simulink model "IC_HW4_Q4"  (R2022b)
settings: Solver=FixedStepAuto  StartTime=0.0  StopTime=SimTime  FixedStep=Delta_t  RelTol=1e-6
values from neighbouring files (symbols this model uses):
  g = 9.81    [aero_guid_dat.m]
  Iyy = 182.5/(Kg2slug*m2ft^2)    (= 247.436636441)    [aero_guid_dat.m]
  L = 0.0065    [aero_guid_dat.m]
undefined symbols (not defined in the file or in its folder): AF, c, Delta_t, Dis, IC, Ixx, Izz, lambda, m, magnitude, N_n, Out_sampleTime, Unc
settings Model: PacingRate=1.400000  Creator=Mahdi  LastModifiedBy=Mahdi
settings OptimizationCC: UseDivisionForNetSlopeComputation=on  GainParamInheritBuiltInType=on  UseFloatMulNetSlope=on  EnhancedBackFolding=on  PassReuseOutputArgsThreshold=0  MaxStackSize=64  OptimizeBlockOrder=speed  DifferentSizesBufferReuse=on
settings DebuggingCC: MultiTaskRateTransMsg=warning  ParameterTunabilityLossMsg=error  UnconnectedInputMsg=warning  UnconnectedOutputMsg=warning  UnconnectedLineMsg=warning
settings ModelReferenceCC: EnableRefExpFcnMdlSchedulingChecks=on
settings SFSimCC: MATLABDynamicMemAlloc=off
settings RTWCC: GenerateReport=on  BuildConfiguration=Faster Runs  LaunchReport=on  DLArmComputeVersion=19.05
settings CodeAppCC: ForceParamTrailComments=on  OperatorAnnotations=on  StateflowObjectComments=on
settings GRTTargetCC: TargetLangStandard=C89/C90 (ANSI)

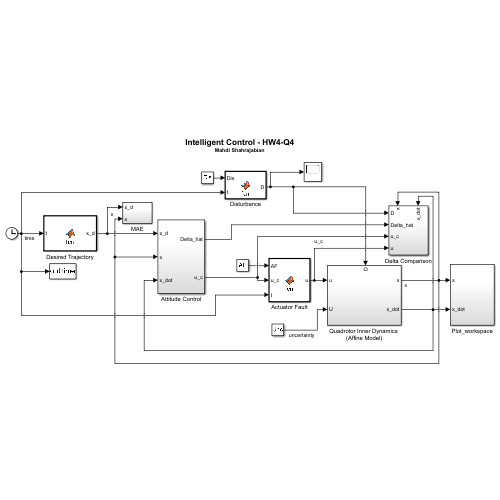
[thumbnail: Simulink's stored preview of the top-level diagram]
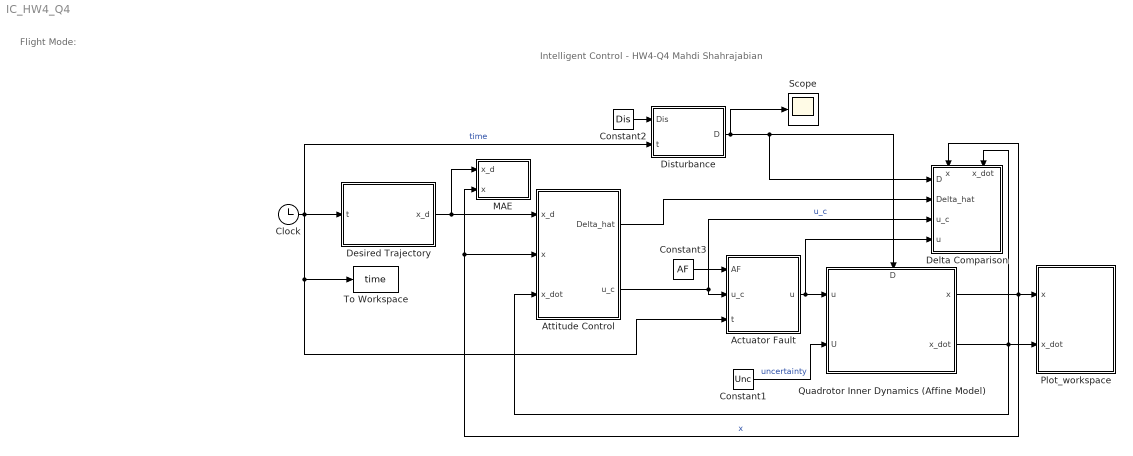
== system IC_HW4_Q4 ==
  note: Flight Mode:
  note: Intelligent Control - HW4-Q4
      | Mahdi Shahrajabian
  Actuator Fault : MATLAB Function  TreatAsAtomicUnit=on
  Attitude Control : Subsystem
  Clock : Clock
  Constant1 : Constant  Value=Unc
  Constant2 : Constant  Value=Dis
  Constant3 : Constant  Value=AF
  Delta Comparison : Subsystem
      settings: PortSchema="{\"entries\":[{\"content\":{\"sides\":[{\"content\":{\"connectorIds\":[\"In1\",\"In2\",\"In3\",\"In4\"]},\"type\":\"ConnectorPlacement.EquallySpacedRectSide\",\"uuid\":\"cdb532f7-5b91-47b5-acb3-9a86cd5c6b77\"},{\"content\":{\"connectorIds\":[],\"side\":\"RIGHT\"},\"type\":\"ConnectorPlacement.EquallySpacedRectSide\",\"uuid\":\"b06da143-48ef-4b64-bdfd-6970dc0cc34f\"},{\"content\":{\"connectorIds\":[\"In5\",\"In6\"],\"side\":\"TOP\"},\"type\":\"ConnectorPlacement.EquallySpacedRectSide\",\"uuid\":\"bf35b783-3952-4033-a28c-7c7593d685ac\"}]},\"type\":\"ConnectorPlacement.EquallySpacedConnector\",\"uuid\":\"8662215e-6394-4b1e-9857-932c5f3d9e43\"}],\"packageUris\":[\"http://schema.mathworks.com/mf0/Connector/R2020b\"],\"version\":\"1.0\"}"
  Desired Trajectory : MATLAB Function  TreatAsAtomicUnit=on
  Disturbance : MATLAB Function  TreatAsAtomicUnit=on
  MAE : Subsystem
  Plot_workspace : Subsystem
  Quadrotor Inner Dynamics (Affine Model) : Subsystem  VariantControl=Choice_1
      settings: PortSchema="{\"entries\":[{\"content\":{\"sides\":[{\"content\":{\"connectorIds\":[\"In1\",\"In2\"]},\"type\":\"ConnectorPlacement.EquallySpacedRectSide\",\"uuid\":\"0e0b7772-be35-4c99-a43c-4efeceea2abb\"},{\"content\":{\"connectorIds\":[\"Out1\",\"Out2\"],\"side\":\"RIGHT\"},\"type\":\"ConnectorPlacement.EquallySpacedRectSide\",\"uuid\":\"5cb7644e-296d-47e5-aec5-64a6e3cb13ec\"},{\"content\":{\"connectorIds\":[\"In3\"],\"side\":\"TOP\"},\"type\":\"ConnectorPlacement.EquallySpacedRectSide\",\"uuid\":\"46b677d2-baa1-4957-a8ea-ecf0c8b5e3e1\"}]},\"type\":\"ConnectorPlacement.EquallySpacedConnector\",\"uuid\":\"4a1aa558-d3d9-4ac2-b56f-16c8e802cec4\"}],\"packageUris\":[\"http://schema.mathworks.com/mf0/Connector/R2020b\"],\"version\":\"1.0\"}"
  Scope : Scope
  To Workspace : ToWorkspace  VariableName=time  SampleTime=Out_sampleTime
      settings: Decimation=5
  wires:
  Quadrotor Inner Dynamics (Affine Model)/2(x_dot) -> Delta Comparison/6(x_dot), Plot_workspace/2(x_dot), Attitude Control/3(x_dot)
  Constant1/1 -> Quadrotor Inner Dynamics (Affine Model)/2(U)  "uncertainty"
  Attitude Control/2(u_c) -> Actuator Fault/2(u_c), Delta Comparison/3(u_c)  "u_c"
  Constant3/1 -> Actuator Fault/1(AF)
  Actuator Fault/1(u) -> Quadrotor Inner Dynamics (Affine Model)/1(u), Delta Comparison/4(u)
  Disturbance/1(D) -> Scope/1, Delta Comparison/1(D), Quadrotor Inner Dynamics (Affine Model)/3(D)
  Attitude Control/1(Delta_hat) -> Delta Comparison/2(Delta_hat)
  Constant2/1 -> Disturbance/1(Dis)
  Desired Trajectory/1(x_d) -> Attitude Control/1(x_d), MAE/1(x_d)
  Clock/1 -> Disturbance/2(t), Actuator Fault/3(t), To Workspace/1, Desired Trajectory/1(t)  "time"
  Quadrotor Inner Dynamics (Affine Model)/1(x) -> MAE/2(x), Attitude Control/2(x), Delta Comparison/5(x), Plot_workspace/1(x)  "x"

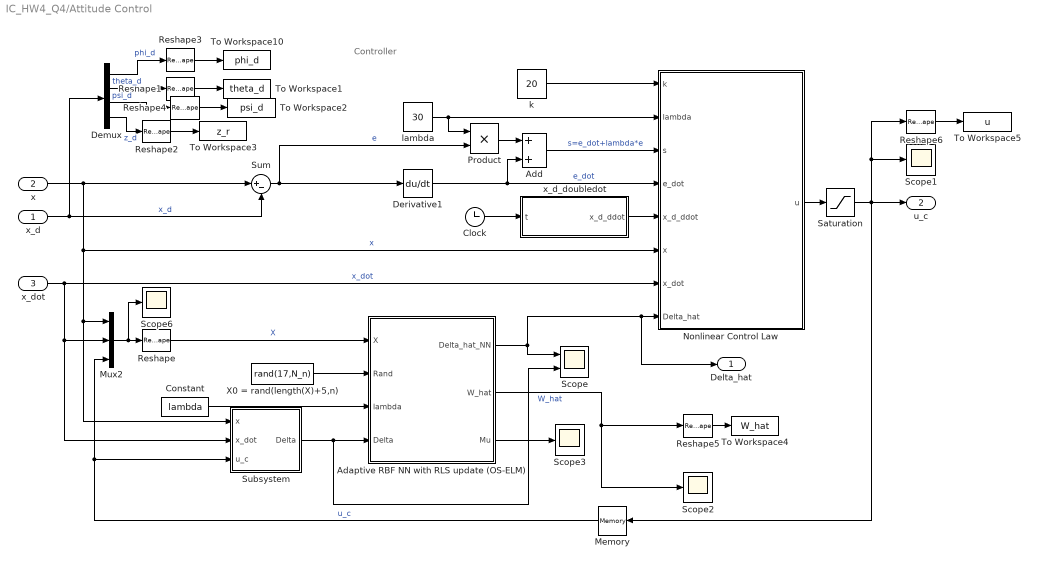
== system IC_HW4_Q4/Attitude Control ==
  note: Controller
  x_d : Inport
  x : Inport  Port=2
  x_dot : Inport  Port=3
  Adaptive RBF NN with RLS update (OS-ELM) : MATLAB Function  TreatAsAtomicUnit=on  SystemSampleTime=0.01
  Add : Sum
  Clock : Clock
  Constant : Constant  Value=lambda
  Demux : Demux
  Derivative1 : Derivative
  Memory : Memory
  Mux2 : Mux  Inputs=3
  Nonlinear Control Law : MATLAB Function  TreatAsAtomicUnit=on  SystemSampleTime=0.01
  Product : Product
  Reshape : Reshape  OutputDimensionality=Column vector (2-D)
  Reshape{1..6} (6 alike) : Reshape
  Saturation : Saturate  UpperLimit=5  LowerLimit=0
  Scope : Scope  NumInputPorts=2
  Scope{1..3,6} (4 alike) : Scope
  Subsystem : Subsystem
  Sum : Sum  Inputs=|+-
  To Workspace1 : ToWorkspace  VariableName=theta_d  SampleTime=Out_sampleTime
      settings: Decimation=5
  To Workspace10 : ToWorkspace  VariableName=phi_d  SampleTime=Out_sampleTime
      settings: Decimation=5
  To Workspace2 : ToWorkspace  VariableName=psi_d  SampleTime=Out_sampleTime
      settings: Decimation=5
  To Workspace3 : ToWorkspace  VariableName=z_r  SampleTime=Out_sampleTime
      settings: Decimation=5
  To Workspace4 : ToWorkspace  VariableName=W_hat  SampleTime=Out_sampleTime
      settings: Decimation=5
  To Workspace5 : ToWorkspace  VariableName=u  SampleTime=Out_sampleTime
      settings: Decimation=5
  X0 = rand(length(X)+5,n) : Constant  Value=rand(17,N_n)
  k : Constant  Value=20
  lambda : Constant  Value=30
  x_d_doubledot : MATLAB Function  TreatAsAtomicUnit=on
  Delta_hat : Outport
  u_c : Outport  Port=2
  wires:
  Nonlinear Control Law/1(u) -> Saturation/1
  x/1 -> Sum/1, Subsystem/1(x), Mux2/1, Nonlinear Control Law/6(x)  "x"
  x_d/1 -> Demux/1, Sum/2  "x_d"
  Sum/1 -> Derivative1/1, Product/2  "e"
  Derivative1/1 -> Add/2, Nonlinear Control Law/4(e_dot)  "e_dot"
  Product/1 -> Add/1
  lambda/1 -> Product/1, Nonlinear Control Law/2(lambda)
  Add/1 -> Nonlinear Control Law/3(s)  "s=e_dot+lambda*e"
  x_dot/1 -> Nonlinear Control Law/7(x_dot), Subsystem/2(x_dot), Mux2/2  "x_dot"
  k/1 -> Nonlinear Control Law/1(k)
  Demux/1 -> Reshape3/1  "phi_d"
  Demux/2 -> Reshape1/1  "theta_d"
  Demux/3 -> Reshape4/1  "psi_d"
  Demux/4 -> Reshape2/1  "z_d"
  Saturation/1 -> Memory/1, Reshape6/1, Scope1/1, u_c/1
  Adaptive RBF NN with RLS update (OS-ELM)/1(Delta_hat_NN) -> Scope/1, Delta_hat/1, Nonlinear Control Law/8(Delta_hat)
  Mux2/1 -> Scope6/1, Reshape/1
  Reshape/1 -> Adaptive RBF NN with RLS update (OS-ELM)/1(X)  "X"
  Memory/1 -> Mux2/3, Subsystem/3(u_c)  "u_c"
  Adaptive RBF NN with RLS update (OS-ELM)/2(W_hat) -> Scope2/1, Reshape5/1  "W_hat"
  X0 = rand(length(X)+5,n)/1 -> Adaptive RBF NN with RLS update (OS-ELM)/2(Rand)
  Reshape3/1 -> To Workspace10/1
  Reshape1/1 -> To Workspace1/1
  Reshape2/1 -> To Workspace3/1
  Reshape4/1 -> To Workspace2/1
  Reshape5/1 -> To Workspace4/1
  Clock/1 -> x_d_doubledot/1(t)
  x_d_doubledot/1(x_d_ddot) -> Nonlinear Control Law/5(x_d_ddot)
  Subsystem/1(Delta) -> Scope/2, Adaptive RBF NN with RLS update (OS-ELM)/4(Delta)
  Constant/1 -> Adaptive RBF NN with RLS update (OS-ELM)/3(lambda)
  Adaptive RBF NN with RLS update (OS-ELM)/3(Mu) -> Scope3/1
  Reshape6/1 -> To Workspace5/1

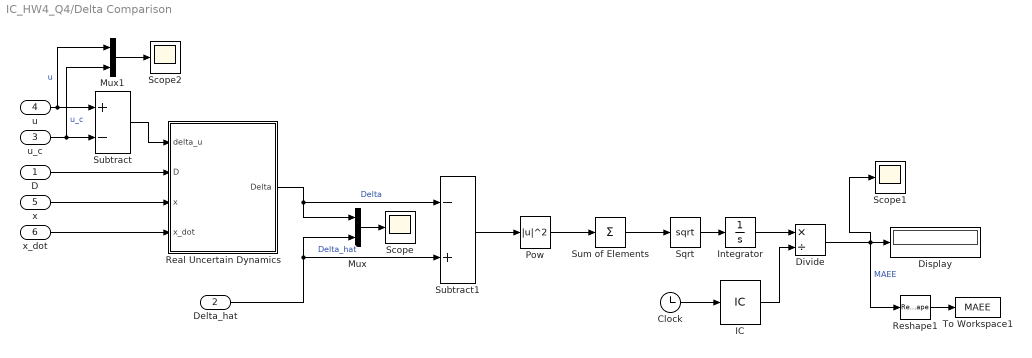
== system IC_HW4_Q4/Delta Comparison ==
  D : Inport
  Delta_hat : Inport  Port=2
  u_c : Inport  Port=3
  u : Inport  Port=4
  x : Inport  Port=5
  x_dot : Inport  Port=6
  Clock : Clock
  Display : Display
  Divide : Product  Inputs=*/
  IC : InitialCondition
  Integrator : Integrator  UpperSaturationLimit=10000  LowerSaturationLimit=-10000
  Mux : Mux  Inputs=2
  Mux1 : Mux  Inputs=2
  Pow : Math  Operator=magnitude^2  RndMeth=Zero
  Real Uncertain Dynamics : MATLAB Function  TreatAsAtomicUnit=on
  Reshape1 : Reshape
  Scope : Scope
  Scope1 : Scope
  Scope2 : Scope
  Sqrt : Sqrt
  Subtract : Sum  Inputs=+-
  Subtract1 : Sum  Inputs=-+
  Sum of Elements : Sum  Inputs=+
  To Workspace1 : ToWorkspace  VariableName=MAEE  SampleTime=-1
      settings: MaxDataPoints=1  Decimation=5
  wires:
  D/1 -> Real Uncertain Dynamics/2(D)
  u_c/1 -> Mux1/2, Subtract/2  "u_c"
  u/1 -> Mux1/1, Subtract/1  "u"
  Subtract/1 -> Real Uncertain Dynamics/1(delta_u)
  Mux/1 -> Scope/1
  x/1 -> Real Uncertain Dynamics/3(x)
  x_dot/1 -> Real Uncertain Dynamics/4(x_dot)
  Delta_hat/1 -> Mux/2, Subtract1/2  "Delta_hat"
  Divide/1 -> Scope1/1, Reshape1/1, Display/1  "MAEE"
  Sqrt/1 -> Integrator/1
  Real Uncertain Dynamics/1(Delta) -> Subtract1/1, Mux/1  "Delta"
  Sum of Elements/1 -> Sqrt/1
  Subtract1/1 -> Pow/1
  Pow/1 -> Sum of Elements/1
  Mux1/1 -> Scope2/1
  Clock/1 -> IC/1
  Integrator/1 -> Divide/1
  Reshape1/1 -> To Workspace1/1
  IC/1 -> Divide/2

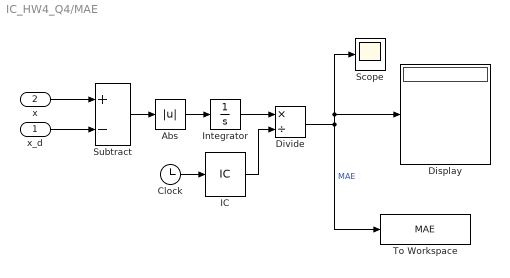
== system IC_HW4_Q4/MAE ==
  x_d : Inport
  x : Inport  Port=2
  Abs : Abs  SaturateOnIntegerOverflow=off
  Clock : Clock
  Display : Display
  Divide : Product  Inputs=*/
  IC : InitialCondition
  Integrator : Integrator
  Scope : Scope
  Subtract : Sum  Inputs=+-
  To Workspace : ToWorkspace  VariableName=MAE  SampleTime=-1
      settings: MaxDataPoints=1
  wires:
  x/1 -> Subtract/1
  x_d/1 -> Subtract/2
  Subtract/1 -> Abs/1
  Abs/1 -> Integrator/1
  Integrator/1 -> Divide/1
  Divide/1 -> Scope/1, Display/1, To Workspace/1  "MAE"
  Clock/1 -> IC/1
  IC/1 -> Divide/2

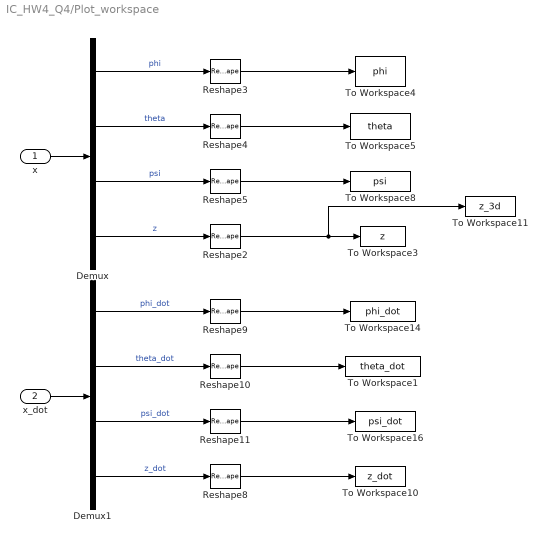
== system IC_HW4_Q4/Plot_workspace ==
  x : Inport
  x_dot : Inport  Port=2
  Demux : Demux
  Demux1 : Demux
  Reshape{2..5,8..11} (8 alike) : Reshape
  To Workspace1 : ToWorkspace  VariableName=theta_dot  SampleTime=Out_sampleTime
      settings: Decimation=5
  To Workspace10 : ToWorkspace  VariableName=z_dot  SampleTime=Out_sampleTime
      settings: Decimation=5
  To Workspace11 : ToWorkspace  VariableName=z_3d  SampleTime=5*Out_sampleTime
      settings: Decimation=5
  To Workspace14 : ToWorkspace  VariableName=phi_dot  SampleTime=Out_sampleTime
      settings: Decimation=5
  To Workspace16 : ToWorkspace  VariableName=psi_dot  SampleTime=Out_sampleTime
      settings: Decimation=5
  To Workspace3 : ToWorkspace  VariableName=z  SampleTime=Out_sampleTime
      settings: Decimation=5
  To Workspace4 : ToWorkspace  VariableName=phi  SampleTime=Out_sampleTime
      settings: Decimation=5
  To Workspace5 : ToWorkspace  VariableName=theta  SampleTime=Out_sampleTime
      settings: Decimation=5
  To Workspace8 : ToWorkspace  VariableName=psi  SampleTime=Out_sampleTime
      settings: Decimation=5
  wires:
  Demux/2 -> Reshape4/1  "theta"
  Demux1/1 -> Reshape9/1  "phi_dot"
  Demux1/4 -> Reshape8/1  "z_dot"
  Demux1/2 -> Reshape10/1  "theta_dot"
  Demux/4 -> Reshape2/1  "z"
  Demux/1 -> Reshape3/1  "phi"
  Demux/3 -> Reshape5/1  "psi"
  Demux1/3 -> Reshape11/1  "psi_dot"
  x/1 -> Demux/1
  Reshape2/1 -> To Workspace11/1, To Workspace3/1
  Reshape3/1 -> To Workspace4/1
  Reshape4/1 -> To Workspace5/1
  Reshape5/1 -> To Workspace8/1
  Reshape8/1 -> To Workspace10/1
  Reshape9/1 -> To Workspace14/1
  Reshape10/1 -> To Workspace1/1
  Reshape11/1 -> To Workspace16/1
  x_dot/1 -> Demux1/1

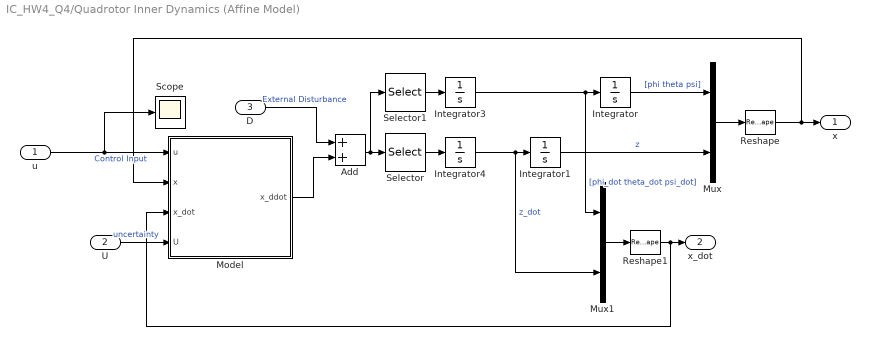
== system IC_HW4_Q4/Quadrotor Inner Dynamics (Affine Model) ==
  u : Inport
  U : Inport  Port=2
  D : Inport  Port=3
  Add : Sum
  Integrator : Integrator  InitialCondition=IC.euler.'  WrapState=on
  Integrator1 : Integrator  InitialCondition=IC.z
  Integrator3 : Integrator  InitialCondition=IC.angRates.'
  Integrator4 : Integrator  InitialCondition=IC.vz
  Model : MATLAB Function  TreatAsAtomicUnit=on
  Mux : Mux  Inputs=2
  Mux1 : Mux  Inputs=2
  Reshape : Reshape  OutputDimensionality=Column vector (2-D)
  Reshape1 : Reshape  OutputDimensionality=Column vector (2-D)
  Scope : Scope
  Selector : Selector  InputPortWidth=4  IndexOptions=Index vector (dialog)  Indices=4  OutputSizes=1
  Selector1 : Selector  InputPortWidth=4  IndexOptions=Index vector (dialog)  Indices=[1 2 3]  OutputSizes=1
  x : Outport
  x_dot : Outport  Port=2
  wires:
  Integrator/1 -> Mux/1  "[phi theta psi]"
  Integrator1/1 -> Mux/2  "z"
  Add/1 -> Selector/1, Selector1/1
  Mux/1 -> Reshape/1
  Selector1/1 -> Integrator3/1
  Integrator3/1 -> Mux1/1, Integrator/1  "[phi_dot theta_dot psi_dot]"
  Selector/1 -> Integrator4/1
  Integrator4/1 -> Mux1/2, Integrator1/1  "z_dot"
  Mux1/1 -> Reshape1/1
  Reshape1/1 -> Model/3(x_dot), x_dot/1
  Reshape/1 -> Model/2(x), x/1
  Model/1(x_ddot) -> Add/2
  D/1 -> Add/1  "External Disturbance"
  U/1 -> Model/4(U)  "uncertainty"
  u/1 -> Scope/1, Model/1(u)  "Control Input"

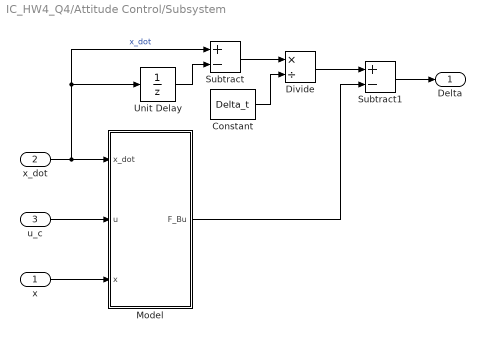
== system IC_HW4_Q4/Attitude Control/Subsystem ==
  x : Inport
  x_dot : Inport  Port=2
  u_c : Inport  Port=3
  Constant : Constant  Value=Delta_t
  Divide : Product  Inputs=*/
  Model : MATLAB Function  TreatAsAtomicUnit=on
  Subtract : Sum  Inputs=+-
  Subtract1 : Sum  Inputs=+-
  Unit Delay : UnitDelay  SampleTime=-1  HasFrameUpgradeWarning=on
  Delta : Outport
  wires:
  Model/1(F_Bu) -> Subtract1/2
  Unit Delay/1 -> Subtract/2
  u_c/1 -> Model/2(u)
  Subtract/1 -> Divide/1
  Constant/1 -> Divide/2
  x_dot/1 -> Unit Delay/1, Subtract/1, Model/1(x_dot)  "x_dot"
  x/1 -> Model/3(x)
  Divide/1 -> Subtract1/1
  Subtract1/1 -> Delta/1

== matlab function IC_HW4_Q4/Delta Comparison/Real Uncertain Dynamics ==
  data: delta_u input; Delta output; D input; x input; x_dot input; m parameter; L parameter; Ixx parameter; Iyy parameter; Izz parameter; c parameter
function Delta = fcn(delta_u,D,x,x_dot, m, L, Ixx, Iyy, Izz, c)
Delta_1 = [x(1)*x(2);
         x_dot(2)*x_dot(3);
         x(1)*x(3);
         0.2*x_dot(4)*x(1)];

B = [0 L/Ixx 0 -L/Ixx;
     -L/Iyy 0 L/Iyy 0;
     c/Izz -c/Izz c/Izz -c/Izz;
     -cos(x(1))*cos(x(2))/m -cos(x(1))*cos(x(2))/m -cos(x(1))*cos(x(2))/m -cos(x(1))*cos(x(2))/m];

Delta = Delta_1 + B*delta_u+D;

== matlab function IC_HW4_Q4/Attitude Control/Adaptive RBF NN with RLS update (OS-ELM) ==
  settings: updateMethod=DISCRETE
  data: X input; Rand input; lambda input; Delta_hat_NN output double size=[4 1]; Delta input; N_n parameter size=1; W_hat output; Mu output
function [Delta_hat_NN,W_hat,Mu]  = fcn(X,Rand,lambda, Delta, N_n)
    X = [X(1);X(2);X(3);X(4)/20;X(5);X(6);X(7);X(8);X(9);X(10);X(11);X(12)]/5;
    n = 12;

    persistent mu
    if isempty(mu)
        mu = zeros(N_n,1); 
    end
   
    X_0 = -1 + 2*Rand(1:n,:);
    sigma = 1.2 + 3*Rand(n+1,:);
    w1_hat = -1 + 2*Rand(n+2,:);
    w2_hat = -1 + 2*Rand(n+3,:);
    w3_hat = -1 + 2*Rand(n+4,:);
    w4_hat = -1 + 2*Rand(n+5,:);

    for i=1:N_n
        mu(i,1) = exp(-(X-X_0(:,i))'*(X-X_0(:,i))/(2*sigma(i)));
    end
    Mu = mu;
    persistent P
    if isempty(P)
        P = 1000*eye(N_n);
    end
    persistent w_1_hat
    if isempty(w_1_hat)
        w_1_hat = w1_hat'; 
    end
    persistent w_2_hat
    if isempty(w_2_hat)
        w_2_hat = w2_hat'; 
    end
    persistent w_3_hat
    if isempty(w_3_hat)
        w_3_hat = w3_hat'; 
    end
    persistent w_4_hat
    if isempty(w_4_hat)
        w_4_hat = w4_hat'; 
    end
    K = P*Mu/(lambda+Mu'*P*Mu);
    % K = P*Mu;
    P = (eye(N_n)-K*Mu')*P/lambda;

    e_1 = Delta(1)-Mu'*w_1_hat;
    e_2 = Delta(2)-Mu'*w_2_hat;
    e_3 = Delta(3)-Mu'*w_3_hat;
    e_4 = Delta(4)-Mu'*w_4_hat;

    w_1_hat = w_1_hat+K*e_1;
    w_2_hat = w_2_hat+K*e_2;
    w_3_hat = w_3_hat+K*e_3;
    w_4_hat = w_4_hat+K*e_4;

    Delta_hat_1 = Mu'*w_1_hat;
    Delta_hat_2 = Mu'*w_2_hat;
    Delta_hat_3 = Mu'*w_3_hat;
    Delta_hat_4 = Mu'*w_4_hat;

    W_hat = [w_1_hat;w_2_hat;w_3_hat;w_4_hat]';
    Delta_hat_NN = [Delta_hat_1;Delta_hat_2;Delta_hat_3;Delta_hat_4];
end

== matlab function IC_HW4_Q4/Attitude Control/Nonlinear Control Law ==
  data: k input; lambda input; s input; e_dot input; x_d_ddot input; x input; x_dot input; u output; g parameter; m parameter; Ixx parameter; Iyy parameter; Izz parameter; L parameter; c parameter; Delta_hat input

function u = fcn(k, lambda, s,e_dot,x_d_ddot,x,x_dot,g, m, Ixx, Iyy, Izz, L, c, Delta_hat)
f = [(Iyy-Izz)*x_dot(2)*x_dot(3)/(Ixx); 
    (Izz-Ixx)*x_dot(1)*x_dot(3)/(Iyy);
    (Ixx-Iyy)*x_dot(1)*x_dot(2)/(Izz);
    g];

B = [0 L/Ixx 0 -L/Ixx;
     -L/Iyy 0 L/Iyy 0;
     c/Izz -c/Izz c/Izz -c/Izz;
     -cos(x(1))*cos(x(2))/m -cos(x(1))*cos(x(2))/m -cos(x(1))*cos(x(2))/m -cos(x(1))*cos(x(2))/m];

u = B\(-f+x_d_ddot-lambda*e_dot-k*s-Delta_hat); % inv(B)*(-f+X_d_ddot-lambda*e_dot-k*s-Delta_hat)
% u = [T1; T2; T3; T4]

== matlab function IC_HW4_Q4/Attitude Control/Subsystem/Model ==
  data: x_dot input; u input size=4; x input; F_Bu output; g parameter; m parameter; Ixx parameter; Iyy parameter; Izz parameter; L parameter; c parameter
function F_Bu  = fcn(x_dot,u,x,g, m, Ixx, Iyy, Izz, L, c)

F = [(Iyy-Izz)*x_dot(2)*x_dot(3)/(Ixx); 
    (Izz-Ixx)*x_dot(1)*x_dot(3)/(Iyy);
    (Ixx-Iyy)*x_dot(1)*x_dot(2)/(Izz);
    g];

% B(X) = [0 L/Ixx 0 -L/Ixx;
%         -L/Iyy 0 L/Iyy 0;
%         c/Izz -c/Izz c/Izz -c/Izz;
%         -cos(phi)*cos(theta)/m -cos(phi)*cos(theta)/m -cos(phi)*cos(theta)/m -cos(phi)*cos(theta)/m]

B = [0 L/Ixx 0 -L/Ixx;
     -L/Iyy 0 L/Iyy 0;
     c/Izz -c/Izz c/Izz -c/Izz;
     -cos(x(1))*cos(x(2))/m -cos(x(1))*cos(x(2))/m -cos(x(1))*cos(x(2))/m -cos(x(1))*cos(x(2))/m];

F_Bu = F+B*u;

== matlab function IC_HW4_Q4/Quadrotor Inner Dynamics (Affine Model)/Model ==
  data: u input size=4; x input; x_dot input; x_ddot output; g parameter; m parameter; Ixx parameter; Iyy parameter; Izz parameter; L parameter; c parameter; U input
function x_ddot  = fcn(u,x,x_dot,g, m, Ixx, Iyy, Izz, L, c, U)
% u = [T1; T2; T3; T4]
% u_in = [F; u_phi; u_theta; u_psi] = T_u*u
% T_u = [1 1 1 1;
%        0 L 0 -L;
%        -L 0 L 0;
%        c -c c -c];
% X = [phi theta psi z]
% X_dot = [phi_dot theta_dot psi_dot z_dot]
% X_ddot = f(X_dot)+B(X)u

% f(X_dot) = [(I_yy-I_zz)*theta_dot*psi_dot/I_xx;
%        (I_zz-I_xx)*phi_dot*psi_dot/I_yy;
%        (I_xx-I_yy)*phi_dot*theta_dot/I_zz;
%        g]

f = [(Iyy-Izz)*x_dot(2)*x_dot(3)/(Ixx); 
    (Izz-Ixx)*x_dot(1)*x_dot(3)/(Iyy);
    (Ixx-Iyy)*x_dot(1)*x_dot(2)/(Izz);
    g];

if U == 1
    Delta_1 = [x(1)*x(2);
             x_dot(2)*x_dot(3);
             x(1)*x(3);
             0.2*x_dot(4)*x(1)];
else
    Delta_1 = zeros(4,1);
end
f = f+Delta_1;
% B(X) = [0 L/Ixx 0 -L/Ixx;
%         -L/Iyy 0 L/Iyy 0;
%         c/Izz -c/Izz c/Izz -c/Izz;
%         -cos(phi)*cos(theta)/m -cos(phi)*cos(theta)/m -cos(phi)*cos(theta)/m -cos(phi)*cos(theta)/m]

B = [0 L/Ixx 0 -L/Ixx;
     -L/Iyy 0 L/Iyy 0;
     c/Izz -c/Izz c/Izz -c/Izz;
     -cos(x(1))*cos(x(2))/m -cos(x(1))*cos(x(2))/m -cos(x(1))*cos(x(2))/m -cos(x(1))*cos(x(2))/m];

x_ddot = f+B*u;

== matlab function IC_HW4_Q4/Actuator Fault ==
  data: AF input; u_c input; u output; t input
function u = fcn(AF,u_c, t)
if AF == 1
    if t<5
        u = u_c;
    elseif t>=5 && t<8
        u = diag([0.8,1,1,1])*u_c;
        % u = diag([0.9,1,1,1])*u_c;
    else
        u = diag([0.8,0.7,1,1])*u_c;
        % u = diag([1,0.9,1,1])*u_c;
    end
else
    u = u_c;
end

== matlab function IC_HW4_Q4/Disturbance ==
  data: Dis input; D output; t input
function D = fcn(Dis, t)
if Dis == 1
    D = [0.05*sin(pi*t/2);
         0.05*sin(pi*t/3);
         0.02*cos(pi*t);
         sin(2*pi*t+pi/6)];
else
    D = zeros(4,1);
end

== matlab function IC_HW4_Q4/Desired Trajectory ==
  data: x_d output; t input
function x_d = fcn(t)
    phi_d = 0.2*sin(pi*t/10);
    theta_d = 0.2*(1-cos(pi*t/15));
    psi_d = 0;
    z_d = 0.5*t;
    x_d = [phi_d;theta_d;psi_d;z_d];
end

== matlab function IC_HW4_Q4/Attitude Control/x_d_doubledot ==
  data: x_d_ddot output; t input
function x_d_ddot = fcn(t)
    phi_d_ddot = -2*pi^2*sin(pi*t/10)/1000;
    theta_d_ddot = 2*pi^2*cos(pi*t/15)/2250;
    psi_d_ddot = 0;
    z_d_ddot = 0;
    x_d_ddot = [phi_d_ddot;theta_d_ddot;psi_d_ddot;z_d_ddot];
end
